simulink model "vehicle_SL"  (R2022a)
settings: Solver=VariableStepAuto  StartTime=0.0  StopTime=20  MaxStep=0.01  RelTol=1e-3
PreLoadFcn:
  | vehicleObject = vehicle.sportSedan;
libraries: SignalEditorBlockLib x1
settings Model: DataDictionary=busObjectsDD.sldd  Creator=grouleau  LastModifiedBy=grouleau

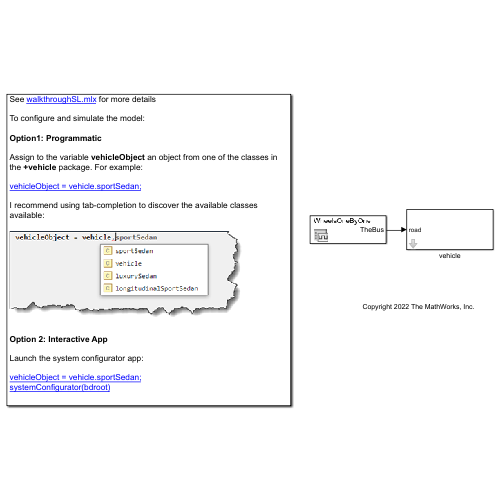
[thumbnail: Simulink's stored preview of the top-level diagram]
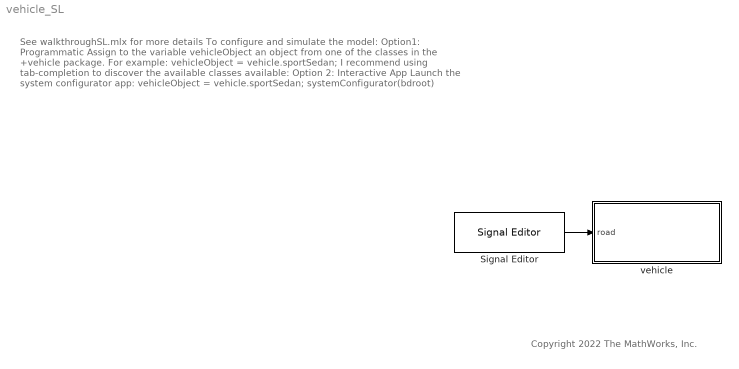
== system vehicle_SL ==
  note: Copyright 2022 The MathWorks, Inc.
  note: See walkthroughSL.mlx for more details
      |
      | To configure and simulate the model:
      |
      | Option1: Programmatic
      |
      | Assign to the variable vehicleObject an object from one of the classes in the +vehicle package. For example:
      |
      | vehicleObject = vehicle.sportSedan;
      |
      | I recommend using tab-completion to discover the available classes available:
      |
      | Option 2: Interactive App
      |
      | Launch the system configurator app:
      |
      | vehicleObject = vehicle.sportSedan;
      | systemConfigurator(bdroot)
  Signal Editor : SignalEditorBlockLib/Signal Editor  FileName=inputProfiles.mat  ActiveScenario=WheelsOneByOne  ActiveSignal=TheBus  IsBus=on  OutputBusObjectStr=Bus: fourWheelsBO  SampleTime=0  Interpolate=off  ZeroCross=off  OutputAfterFinalValue=Setting to zero  Unit=inherit  PreserveSignalName=on
  vehicle : Subsystem  mask(slPart){obj=vehicleObject}
      mask prompts: obj "slPart Object:"
      mask help: This subsystem implements a simplified vehicle and its suspension. To configure the vehicle, assign an object instantiated from one of the class in the "+vehicle" folder.
      mask init:
      | obj.maskInit(gcb);
      mask DialogControl Control3 Prompt: See walkthroughSL.mlx for more examples
      mask DialogControl Control3 Callback: open('walkthroughSL.mlx')
      mask DialogControl Container3 Prompt: Example
      mask DialogControl Control2 Prompt: vehicleObject = vehicle.sportSedan;
      mask DialogControl Control2 Callback: vehicleObject = vehicle.sportSedan;
  wires:
  Signal Editor/1 -> vehicle/1(road)

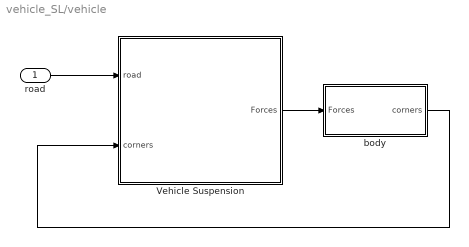
== system vehicle_SL/vehicle ==
  road : Inport
  Vehicle Suspension : Subsystem  AncestorBlock=suspensionLib/Vehicel Suspension  Variant=on  VariantControlMode=label  LabelModeActiveChoice=suspension.threeDof  mask(slPart){obj=obj.Suspension}
      mask prompts: obj "slPart Object:"
      mask help: Container block for all slPart blocks
      mask init:
      | obj.maskInit(gcb);
  body : Subsystem  mask(slPart){obj=obj.Body}
      mask prompts: obj "slPart Object:"
      mask help: Container block for all slPart blocks
      mask init:
      | obj.maskInit(gcb);
  wires:
  Vehicle Suspension/1(Forces) -> body/1(Forces)
  body/1(corners) -> Vehicle Suspension/2(corners)
  road/1 -> Vehicle Suspension/1(road)

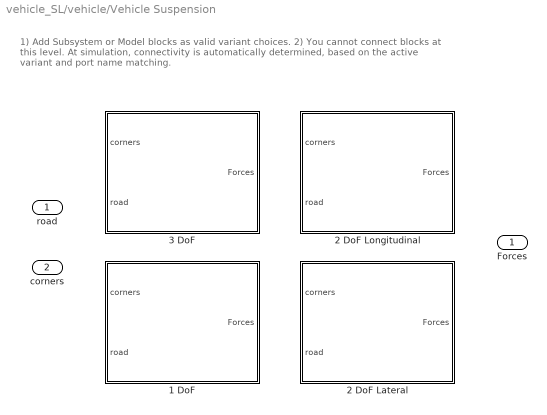
== system vehicle_SL/vehicle/Vehicle Suspension ==
  note: 1) Add Subsystem or Model blocks as valid variant choices.
      | 2) You cannot connect blocks at this level. At simulation, connectivity is automatically
      | determined, based on the active variant and port name matching.
  road : Inport
  corners : Inport  Port=2
  1 DoF : Subsystem  VariantControl=suspension.oneDof
  2 DoF Lateral : Subsystem  VariantControl=suspension.twoDofLateral
  2 DoF Longitudinal : Subsystem  VariantControl=suspension.twoDofLongitudinal
  3 DoF : Subsystem  VariantControl=suspension.threeDof
  Forces : Outport

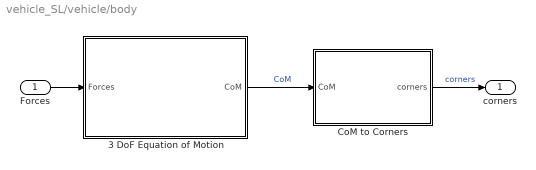
== system vehicle_SL/vehicle/body ==
  Forces : Inport
  3 DoF Equation of Motion : Subsystem
  CoM to Corners : Subsystem
  corners : Outport
  wires:
  3 DoF Equation of Motion/1(CoM) -> CoM to Corners/1(CoM)  "CoM"
  Forces/1 -> 3 DoF Equation of Motion/1(Forces)
  CoM to Corners/1(corners) -> corners/1  "corners"

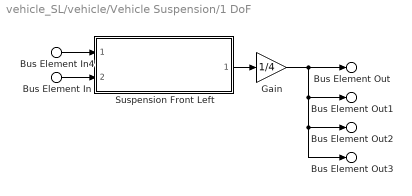
== system vehicle_SL/vehicle/Vehicle Suspension/1 DoF ==
  Bus Element In : Inport  PortName=corners  Element=FrontLeft
  Bus Element In4 : Inport  Port=2  PortName=road  Element=FrontLeft
  Gain : Gain  Gain=1/4
  Suspension Front Left : Subsystem  ReferencedSubsystem=suspension_ss  obj=obj.Suspension
      settings: AttributesFormatString=%<obj>
  Bus Element Out : Outport  PortName=Forces  Element=FrontLeft
  Bus Element Out1 : Outport  PortName=Forces  Element=FrontRight
  Bus Element Out2 : Outport  PortName=Forces  Element=RearLeft
  Bus Element Out3 : Outport  PortName=Forces  Element=RearRight
  wires:
  Bus Element In4/1 -> Suspension Front Left/1
  Bus Element In/1 -> Suspension Front Left/2
  Suspension Front Left/1 -> Gain/1
  Gain/1 -> Bus Element Out3/1, Bus Element Out2/1, Bus Element Out1/1, Bus Element Out/1

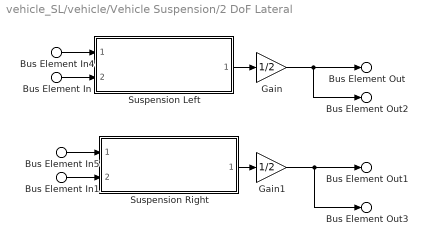
== system vehicle_SL/vehicle/Vehicle Suspension/2 DoF Lateral ==
  Bus Element In : Inport  PortName=corners  Element=FrontLeft
  Bus Element In1 : Inport  PortName=corners  Element=FrontRight
  Bus Element In4 : Inport  Port=2  PortName=road  Element=FrontLeft
  Bus Element In5 : Inport  Port=2  PortName=road  Element=FrontRight
  Gain : Gain  Gain=1/2
  Gain1 : Gain  Gain=1/2
  Suspension Left : Subsystem  ReferencedSubsystem=suspension_ss  obj=obj.Left
      settings: AttributesFormatString=%<obj>
  Suspension Right : Subsystem  ReferencedSubsystem=suspension_ss  obj=obj.Right
      settings: AttributesFormatString=%<obj>
  Bus Element Out : Outport  PortName=Forces  Element=FrontLeft
  Bus Element Out1 : Outport  PortName=Forces  Element=FrontRight
  Bus Element Out2 : Outport  PortName=Forces  Element=RearLeft
  Bus Element Out3 : Outport  PortName=Forces  Element=RearRight
  wires:
  Bus Element In5/1 -> Suspension Right/1
  Bus Element In4/1 -> Suspension Left/1
  Bus Element In1/1 -> Suspension Right/2
  Bus Element In/1 -> Suspension Left/2
  Suspension Right/1 -> Gain1/1
  Suspension Left/1 -> Gain/1
  Gain/1 -> Bus Element Out2/1, Bus Element Out/1
  Gain1/1 -> Bus Element Out3/1, Bus Element Out1/1

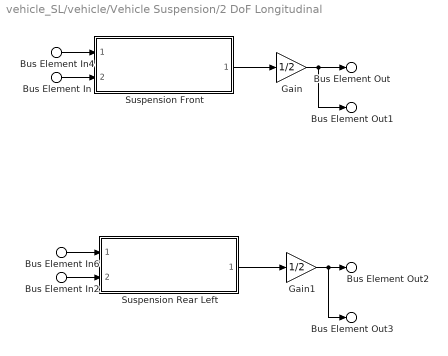
== system vehicle_SL/vehicle/Vehicle Suspension/2 DoF Longitudinal ==
  Bus Element In : Inport  PortName=corners  Element=FrontLeft
  Bus Element In2 : Inport  PortName=corners  Element=RearLeft
  Bus Element In4 : Inport  Port=2  PortName=road  Element=FrontLeft
  Bus Element In6 : Inport  Port=2  PortName=road  Element=RearLeft
  Gain : Gain  Gain=1/2
  Gain1 : Gain  Gain=1/2
  Suspension Front : Subsystem  ReferencedSubsystem=suspension_ss  obj=obj.Front
      settings: AttributesFormatString=%<obj>
  Suspension Rear Left : Subsystem  ReferencedSubsystem=suspension_ss  obj=obj.Rear
      settings: AttributesFormatString=%<obj>
  Bus Element Out : Outport  PortName=Forces  Element=FrontLeft
  Bus Element Out1 : Outport  PortName=Forces  Element=FrontRight
  Bus Element Out2 : Outport  PortName=Forces  Element=RearLeft
  Bus Element Out3 : Outport  PortName=Forces  Element=RearRight
  wires:
  Bus Element In6/1 -> Suspension Rear Left/1
  Bus Element In4/1 -> Suspension Front/1
  Bus Element In2/1 -> Suspension Rear Left/2
  Bus Element In/1 -> Suspension Front/2
  Suspension Front/1 -> Gain/1
  Gain/1 -> Bus Element Out1/1, Bus Element Out/1
  Suspension Rear Left/1 -> Gain1/1
  Gain1/1 -> Bus Element Out3/1, Bus Element Out2/1

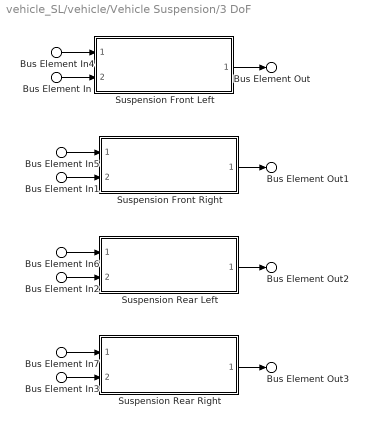
== system vehicle_SL/vehicle/Vehicle Suspension/3 DoF ==
  Bus Element In : Inport  PortName=corners  Element=FrontLeft
  Bus Element In1 : Inport  PortName=corners  Element=FrontRight
  Bus Element In2 : Inport  PortName=corners  Element=RearLeft
  Bus Element In3 : Inport  PortName=corners  Element=RearRight
  Bus Element In4 : Inport  Port=2  PortName=road  Element=FrontLeft
  Bus Element In5 : Inport  Port=2  PortName=road  Element=FrontRight
  Bus Element In6 : Inport  Port=2  PortName=road  Element=RearLeft
  Bus Element In7 : Inport  Port=2  PortName=road  Element=RearRight
  Suspension Front Left : Subsystem  ReferencedSubsystem=suspension_ss  obj=obj.FrontLeft
      settings: AttributesFormatString=%<obj>
  Suspension Front Right : Subsystem  ReferencedSubsystem=suspension_ss  obj=obj.FrontRight
      settings: AttributesFormatString=%<obj>
  Suspension Rear Left : Subsystem  ReferencedSubsystem=suspension_ss  obj=obj.RearLeft
      settings: AttributesFormatString=%<obj>
  Suspension Rear Right : Subsystem  ReferencedSubsystem=suspension_ss  obj=obj.RearRight
      settings: AttributesFormatString=%<obj>
  Bus Element Out : Outport  PortName=Forces  Element=FrontLeft
  Bus Element Out1 : Outport  PortName=Forces  Element=FrontRight
  Bus Element Out2 : Outport  PortName=Forces  Element=RearLeft
  Bus Element Out3 : Outport  PortName=Forces  Element=RearRight
  wires:
  Suspension Rear Left/1 -> Bus Element Out2/1
  Suspension Rear Right/1 -> Bus Element Out3/1
  Suspension Front Left/1 -> Bus Element Out/1
  Suspension Front Right/1 -> Bus Element Out1/1
  Bus Element In/1 -> Suspension Front Left/2
  Bus Element In1/1 -> Suspension Front Right/2
  Bus Element In2/1 -> Suspension Rear Left/2
  Bus Element In3/1 -> Suspension Rear Right/2
  Bus Element In4/1 -> Suspension Front Left/1
  Bus Element In5/1 -> Suspension Front Right/1
  Bus Element In6/1 -> Suspension Rear Left/1
  Bus Element In7/1 -> Suspension Rear Right/1

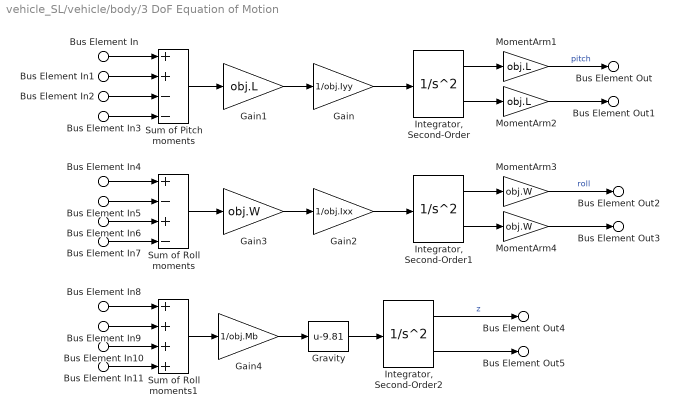
== system vehicle_SL/vehicle/body/3 DoF Equation of Motion ==
  Bus Element In : Inport  PortName=Forces  Element=FrontLeft
  Bus Element In4 : Inport  PortName=Forces  Element=FrontLeft
  Bus Element In8 : Inport  PortName=Forces  Element=FrontLeft
  Bus Element In1 : Inport  PortName=Forces  Element=FrontRight
  Bus Element In5 : Inport  PortName=Forces  Element=FrontRight
  Bus Element In9 : Inport  PortName=Forces  Element=FrontRight
  Bus Element In2 : Inport  PortName=Forces  Element=RearLeft
  Bus Element In6 : Inport  PortName=Forces  Element=RearLeft
  Bus Element In10 : Inport  PortName=Forces  Element=RearLeft
  Bus Element In3 : Inport  PortName=Forces  Element=RearRight
  Bus Element In7 : Inport  PortName=Forces  Element=RearRight
  Bus Element In11 : Inport  PortName=Forces  Element=RearRight
  Gain : Gain  Gain=1/obj.Iyy
  Gain1 : Gain  Gain=obj.L
  Gain2 : Gain  Gain=1/obj.Ixx
  Gain3 : Gain  Gain=obj.W
  Gain4 : Gain  Gain=1/obj.Mb
  Gravity : Bias  Bias=-9.81  SaturateOnIntegerOverflow=off
  "Integrator, Second-Order" : SecondOrderIntegrator
  "Integrator, Second-Order1" : SecondOrderIntegrator
  "Integrator, Second-Order2" : SecondOrderIntegrator
  MomentArm1 : Gain  Gain=obj.L  SaturateOnIntegerOverflow=on  OutDataTypeStr=Inherit: Same as input  ParamDataTypeStr=Inherit: Same as input
  MomentArm2 : Gain  Gain=obj.L  SaturateOnIntegerOverflow=on  OutDataTypeStr=Inherit: Same as input  ParamDataTypeStr=Inherit: Same as input
  MomentArm3 : Gain  Gain=obj.W  SaturateOnIntegerOverflow=on  OutDataTypeStr=Inherit: Same as input  ParamDataTypeStr=Inherit: Same as input
  MomentArm4 : Gain  Gain=obj.W  SaturateOnIntegerOverflow=on  OutDataTypeStr=Inherit: Same as input  ParamDataTypeStr=Inherit: Same as input
  Sum of Pitch moments : Sum  Inputs=++--
  Sum of Roll moments : Sum  Inputs=+-+-
  Sum of Roll moments1 : Sum  Inputs=++++
  Bus Element Out : Outport  PortName=CoM  Element=pitch
  Bus Element Out1 : Outport  PortName=CoM  Element=pitchRate
  Bus Element Out2 : Outport  PortName=CoM  Element=roll
  Bus Element Out3 : Outport  PortName=CoM  Element=rollRate
  Bus Element Out4 : Outport  PortName=CoM  Element=z
  Bus Element Out5 : Outport  PortName=CoM  Element=zDot
  wires:
  "Integrator, Second-Order"/2 -> MomentArm2/1
  Bus Element In3/1 -> Sum of Pitch moments/4
  Gain1/1 -> Gain/1
  Sum of Roll moments1/1 -> Gain4/1
  "Integrator, Second-Order1"/1 -> MomentArm3/1
  Bus Element In/1 -> Sum of Pitch moments/1
  "Integrator, Second-Order1"/2 -> MomentArm4/1
  Bus Element In1/1 -> Sum of Pitch moments/2
  Bus Element In2/1 -> Sum of Pitch moments/3
  Bus Element In7/1 -> Sum of Roll moments/4
  Bus Element In6/1 -> Sum of Roll moments/3
  Gain2/1 -> "Integrator, Second-Order1"/1
  Bus Element In5/1 -> Sum of Roll moments/2
  Gain3/1 -> Gain2/1
  Sum of Roll moments/1 -> Gain3/1
  Sum of Pitch moments/1 -> Gain1/1
  Gain4/1 -> Gravity/1
  Bus Element In10/1 -> Sum of Roll moments1/3
  Bus Element In9/1 -> Sum of Roll moments1/2
  Gain/1 -> "Integrator, Second-Order"/1
  "Integrator, Second-Order"/1 -> MomentArm1/1
  "Integrator, Second-Order2"/2 -> Bus Element Out5/1
  Bus Element In11/1 -> Sum of Roll moments1/4
  "Integrator, Second-Order2"/1 -> Bus Element Out4/1  "z"
  Bus Element In4/1 -> Sum of Roll moments/1
  Bus Element In8/1 -> Sum of Roll moments1/1
  MomentArm1/1 -> Bus Element Out/1  "pitch"
  MomentArm2/1 -> Bus Element Out1/1
  MomentArm3/1 -> Bus Element Out2/1  "roll"
  MomentArm4/1 -> Bus Element Out3/1
  Gravity/1 -> "Integrator, Second-Order2"/1

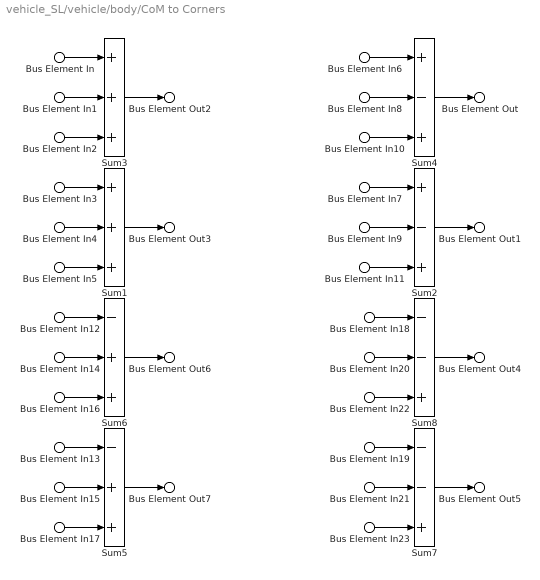
== system vehicle_SL/vehicle/body/CoM to Corners ==
  Bus Element In{,6,12,18} (4 alike) : Inport  PortName=CoM  Element=pitch
  Bus Element In{1,8,14,20} (4 alike) : Inport  PortName=CoM  Element=roll
  Bus Element In{2,10,16,22} (4 alike) : Inport  PortName=CoM  Element=z
  Bus Element In{3,7,13,19} (4 alike) : Inport  PortName=CoM  Element=pitchRate
  Bus Element In{4,9,15,21} (4 alike) : Inport  PortName=CoM  Element=rollRate
  Bus Element In{5,11,17,23} (4 alike) : Inport  PortName=CoM  Element=zDot
  Sum1 : Sum  Inputs=+++  InputSameDT=on  SaturateOnIntegerOverflow=on  OutDataTypeStr=Inherit: Same as first input
  Sum2 : Sum  Inputs=+-+  InputSameDT=on  SaturateOnIntegerOverflow=on  OutDataTypeStr=Inherit: Same as first input
  Sum3 : Sum  Inputs=+++  InputSameDT=on  SaturateOnIntegerOverflow=on  OutDataTypeStr=Inherit: Same as first input
  Sum4 : Sum  Inputs=+-+  InputSameDT=on  SaturateOnIntegerOverflow=on  OutDataTypeStr=Inherit: Same as first input
  Sum5 : Sum  Inputs=-++  InputSameDT=on  SaturateOnIntegerOverflow=on  OutDataTypeStr=Inherit: Same as first input
  Sum6 : Sum  Inputs=-++  InputSameDT=on  SaturateOnIntegerOverflow=on  OutDataTypeStr=Inherit: Same as first input
  Sum7 : Sum  Inputs=--+  InputSameDT=on  SaturateOnIntegerOverflow=on  OutDataTypeStr=Inherit: Same as first input
  Sum8 : Sum  Inputs=--+  InputSameDT=on  SaturateOnIntegerOverflow=on  OutDataTypeStr=Inherit: Same as first input
  Bus Element Out2 : Outport  PortName=corners  Element=FrontLeft.z
  Bus Element Out3 : Outport  PortName=corners  Element=FrontLeft.zDot
  Bus Element Out6 : Outport  PortName=corners  Element=RearLeft.z
  Bus Element Out7 : Outport  PortName=corners  Element=RearLeft.zDot
  Bus Element Out : Outport  PortName=corners  Element=FrontRight.z
  Bus Element Out1 : Outport  PortName=corners  Element=FrontRight.zDot
  Bus Element Out4 : Outport  PortName=corners  Element=RearRight.z
  Bus Element Out5 : Outport  PortName=corners  Element=RearRight.zDot
  wires:
  Bus Element In/1 -> Sum3/1
  Bus Element In1/1 -> Sum3/2
  Bus Element In2/1 -> Sum3/3
  Sum3/1 -> Bus Element Out2/1
  Bus Element In5/1 -> Sum1/3
  Bus Element In4/1 -> Sum1/2
  Bus Element In3/1 -> Sum1/1
  Sum1/1 -> Bus Element Out3/1
  Bus Element In7/1 -> Sum2/1
  Bus Element In9/1 -> Sum2/2
  Bus Element In11/1 -> Sum2/3
  Bus Element In10/1 -> Sum4/3
  Bus Element In8/1 -> Sum4/2
  Bus Element In6/1 -> Sum4/1
  Sum4/1 -> Bus Element Out/1
  Sum2/1 -> Bus Element Out1/1
  Bus Element In13/1 -> Sum5/1
  Bus Element In15/1 -> Sum5/2
  Bus Element In17/1 -> Sum5/3
  Bus Element In16/1 -> Sum6/3
  Bus Element In14/1 -> Sum6/2
  Bus Element In12/1 -> Sum6/1
  Sum6/1 -> Bus Element Out6/1
  Sum5/1 -> Bus Element Out7/1
  Bus Element In18/1 -> Sum8/1
  Bus Element In20/1 -> Sum8/2
  Bus Element In22/1 -> Sum8/3
  Bus Element In23/1 -> Sum7/3
  Bus Element In21/1 -> Sum7/2
  Bus Element In19/1 -> Sum7/1
  Sum8/1 -> Bus Element Out4/1
  Sum7/1 -> Bus Element Out5/1
